simulink model "aspa_2w_towed"  (R2016a)
settings: Solver=VariableStepAuto  StartTime=0.0  StopTime=100  RelTol=1e-3
undefined symbols (not defined in the file): b1, b2, I, k1, k2, k3, k4, LF, LR, M_sb, M_UsbF, M_UsbR
libraries: simulink x2
settings Model: Creator=mm395  LastModifiedBy=mm395
settings GRTTargetCC: GeneratePreprocessorConditionals=Use local settings

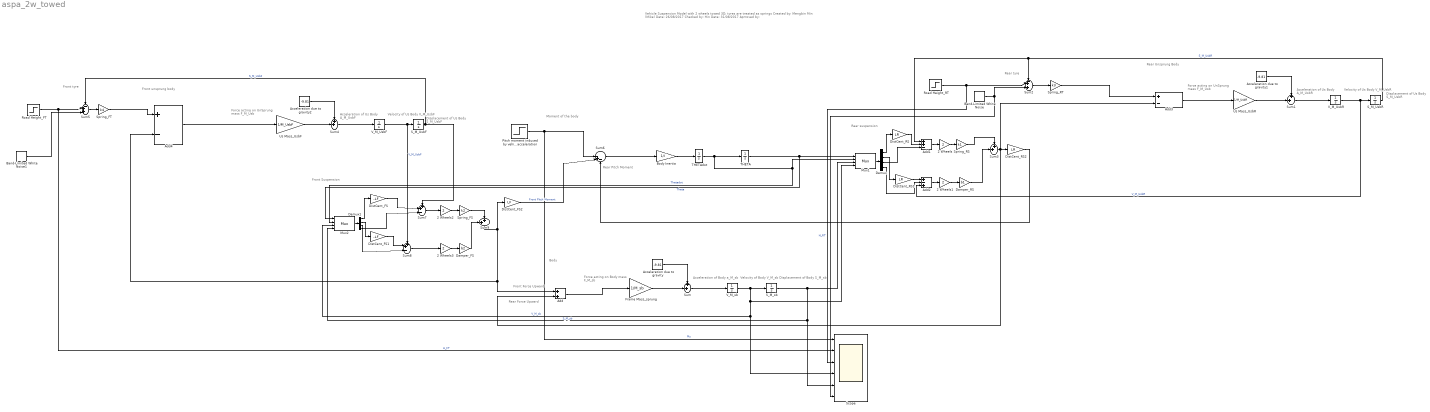
== system aspa_2w_towed ==
  note: Front tyre
  note: Rear tyre
  note: Moment of the body
  note: Rear Force Upward
  note: Front Force Upward
  note: Rear Pitch Moment
  note: Body
  note: Front Suspension
  note: Front unsprung body
  note: Rear Unsprung Body
  note: Acceleration of Body
      | a_M_sb
  note: Force acting on Body mass
      | F_M_sb
  note: Velocity of Body
      | V_M_sb
  note: Displacement of Body
      | S_M_sb
  note: Rear suspension
  note: Acceleration of Us Body
      | A_M_UsbR
  note: Force acting on UnSprung mass
      | F_M_Usb
  note: Velocity of Us Body
      | V_M_UsbR
  note: Displacement of Us Body
      | S_M_UsbR
  note: Acceleration of Us Body
      | A_M_UsbF
  note: Force acting on UnSprung mass
      | F_M_Usb
  note: Velocity of Us Body
      | V_M_UsbF
  note: Displacement of Us Body
      | S_M_UsbF
  note: Vehicle Suspension Model with 2 wheels towed
      | 3D; tyres are treated as springs
      | Created by: Mengbin Min (Mike) Date: 26/08/2017
      | Checked by: Hin Date: 31/08/2017
      | Aprroved by:
  2 Wheels{,1..3} (4 alike) : Gain  Gain=2
  Acceleration due to gravity : Constant  Value=-9.81
  Acceleration due to gravity1 : Constant  Value=-9.81
  Acceleration due to gravity2 : Constant  Value=-9.81
  Add : Sum
  Add1 : Sum  Inputs=++-
  Add2 : Sum  Inputs=+-+
  Add3 : Sum  Inputs=+-
  Add4 : Sum  Inputs=+-
  Band-Limited White Noise : simulink/Sources/Band-Limited White Noise  Cov=[0.0001]  Ts=0.1  seed=[23341]
  Band-Limited White Noise1 : simulink/Sources/Band-Limited White Noise  Cov=[0.0001]  Ts=0.1  seed=[23341]
  Body Inertia : Gain  Gain=1/I  SaturateOnIntegerOverflow=on  OutDataTypeStr=Inherit: Same as input  ParamDataTypeStr=Inherit: Same as input
  Damper_FS : Gain  Gain=b2
  Damper_RS : Gain  Gain=b1
  Demux : Demux
  Demux1 : Demux
  DistCent_FS : Gain  Gain=-LF
  DistCent_FS1 : Gain  Gain=-LF
  DistCent_FS2 : Gain  Gain=LF
  DistCent_RS : Gain  Gain=LR
  DistCent_RS1 : Gain  Gain=LR
  DistCent_RS2 : Gain  Gain=LR
  Frame Mass_sprung : Gain  Gain=1/M_sb
  Mux1 : Mux
      settings: DisplayOption=signals
  Mux2 : Mux
      settings: DisplayOption=signals
  Pitch moment induced by vehicle acceleration : Step  After=100  SampleTime=0
  Road Height_FT : Step  Time=2  After=0  SampleTime=0
  Road Height_RT : Step  Time=4  After=0  SampleTime=0
  S_M_UsbF : Integrator
  S_M_UsbR : Integrator
  S_M_sb : Integrator
  Scope : Scope  NumInputPorts=6
  Spring_FS : Gain  Gain=k2
  Spring_FT : Gain  Gain=k4
  "Spring_RS " : Gain  Gain=k1
  Spring_RT : Gain  Gain=k3
  Sum{,1,3..4,9} (5 alike) : Sum  Inputs=++|
  Sum2 : Sum  Inputs=-++|
  Sum5 : Sum  Inputs=-++|
  Sum6 : Sum  Inputs=||-+-  SaturateOnIntegerOverflow=on  InputSameDT=on  OutDataTypeStr=Inherit: Same as first input
  Sum7 : Sum  Inputs=++-|
  Sum8 : Sum  Inputs=++-|
  THETA : Integrator  InitialCondition=-8.7e-20
  THETAdot : Integrator  InitialCondition=8.04e-28
  Us Mass_UsbF : Gain  Gain=1/M_UsbF
  Us Mass_UsbR : Gain  Gain=1/M_UsbR
  V_M_UsbF : Integrator
  V_M_UsbR : Integrator
  V_M_sb : Integrator
  wires:
  Add/1 -> Frame Mass_sprung/1
  Frame Mass_sprung/1 -> Sum/2
  Acceleration due to gravity/1 -> Sum/1
  V_M_sb/1 -> Scope/4, Mux2/3, Mux1/4, S_M_sb/1  "V_M_sb"
  S_M_sb/1 -> Scope/5, Mux2/4, Mux1/3  "S_M_sb"
  Mux1/1 -> Demux/1
  Sum/1 -> V_M_sb/1
  Pitch moment induced by vehicle acceleration/1 -> Scope/1, Sum6/1  "My"
  Sum6/1 -> Body Inertia/1
  DistCent_RS/1 -> Add1/2
  DistCent_FS2/1 -> Sum6/2  "Front Pitch Moment"
  Body Inertia/1 -> THETAdot/1
  THETA/1 -> Mux2/1, Mux1/1  "Theta"
  THETAdot/1 -> Mux2/2, Mux1/2, THETA/1  "Thetadot"
  Demux/3 -> Add1/3
  Demux/1 -> DistCent_RS/1
  Damper_RS/1 -> Sum3/2
  Damper_FS/1 -> Sum9/1
  Spring_FS/1 -> Sum9/2
  Mux2/1 -> Demux1/1
  Demux1/3 -> Sum8/3
  Demux1/1 -> DistCent_FS/1
  Demux/2 -> DistCent_RS1/1
  DistCent_RS1/1 -> Add2/1
  Demux/4 -> Add2/2
  Add3/1 -> Us Mass_UsbR/1
  Us Mass_UsbR/1 -> Sum1/2
  Acceleration due to gravity1/1 -> Sum1/1
  V_M_UsbR/1 -> Add2/3, S_M_UsbR/1  "V_M_UsbR"
  Sum1/1 -> V_M_UsbR/1
  S_M_UsbR/1 -> Sum2/1, Add1/1  "S_M_UsbR"
  "Spring_RS "/1 -> Sum3/1
  Road Height_RT/1 -> Scope/3, Sum2/2  "H_RT"
  Sum2/1 -> Spring_RT/1
  Spring_RT/1 -> Add3/1
  Add4/1 -> Us Mass_UsbF/1
  Us Mass_UsbF/1 -> Sum4/2
  Acceleration due to gravity2/1 -> Sum4/1
  V_M_UsbF/1 -> Sum8/1, S_M_UsbF/1  "V_M_UsbF"
  Sum4/1 -> V_M_UsbF/1
  S_M_UsbF/1 -> Sum7/1, Sum5/1  "S_M_UsbF"
  Road Height_FT/1 -> Scope/2, Sum5/2  "H_FT"
  Sum5/1 -> Spring_FT/1
  Spring_FT/1 -> Add4/1
  DistCent_RS2/1 -> Sum6/3
  Demux1/4 -> Sum7/3
  DistCent_FS/1 -> Sum7/2
  Sum7/1 -> 2 Wheels2/1
  Demux1/2 -> DistCent_FS1/1
  DistCent_FS1/1 -> Sum8/2
  Sum8/1 -> 2 Wheels3/1
  Sum9/1 -> DistCent_FS2/1, Add4/2, Add/1
  Add1/1 -> 2 Wheels/1
  2 Wheels/1 -> "Spring_RS "/1
  2 Wheels1/1 -> Damper_RS/1
  Add2/1 -> 2 Wheels1/1
  2 Wheels2/1 -> Spring_FS/1
  2 Wheels3/1 -> Damper_FS/1
  Sum3/1 -> Add/2, DistCent_RS2/1, Add3/2
  Band-Limited White Noise1/1 -> Sum5/3
  Band-Limited White Noise/1 -> Sum2/3, Scope/6
